simulink model "perturbacion2"  (R2018b)
settings: Solver=VariableStepAuto  StartTime=0.0  StopTime=10.0  RelTol=1e-3
undefined symbols (not defined in the file): AHat, BHat, CHat, DHat, FHat, K, Kgain, Tao
settings Model: Creator=AlfredoMaussa  LastModifiedBy=AlfredoMaussa
settings SolverCC: ZeroCrossAlgorithm=Adaptive
settings DebuggingCC: IgnoredZcDiagnostic=none

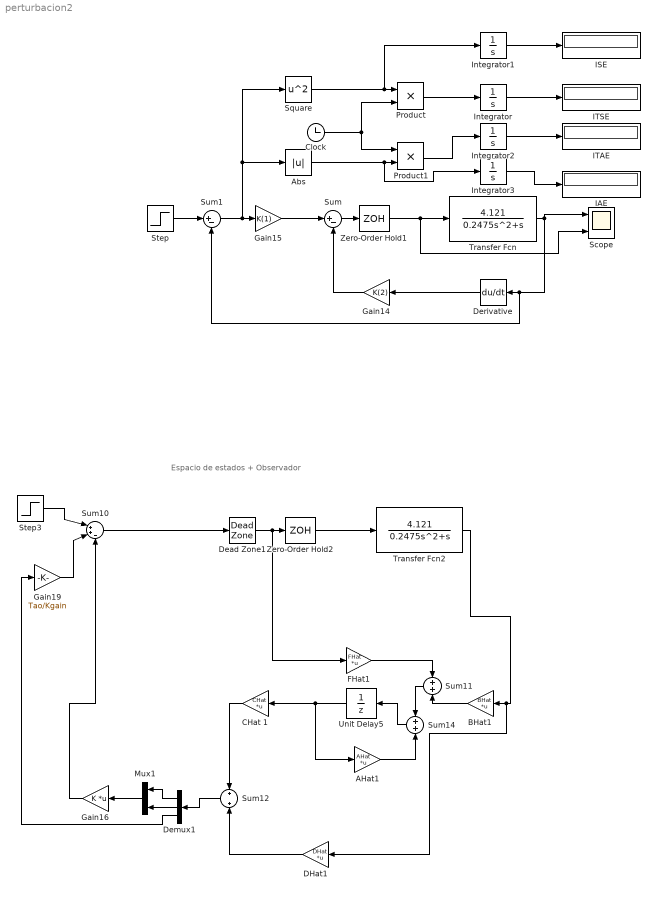
== system perturbacion2 ==
  note: Espacio de estados + Observador
  AHat1 : Gain  Gain=AHat  Multiplication=Matrix(K*u)
  Abs : Abs
  BHat1 : Gain  Gain=BHat  Multiplication=Matrix(K*u)
  CHat 1 : Gain  Gain=CHat  Multiplication=Matrix(K*u)
  Clock : Clock
  DHat1 : Gain  Gain=DHat  Multiplication=Matrix(K*u)
  Dead Zone1 : DeadZone  LowerValue=0  UpperValue=0  SaturateOnIntegerOverflow=on
  Demux1 : Demux  Outputs=3
  Derivative : Derivative  CoefficientInTFapproximation=100
  FHat1 : Gain  Gain=FHat  Multiplication=Matrix(K*u)
  Gain14 : Gain  Gain=K(2)
  Gain15 : Gain  Gain=K(1)
  Gain16 : Gain  Gain=K  Multiplication=Matrix(K*u)
  Gain19 : Gain  Gain=Tao/Kgain
  IAE : Display
  ISE : Display
  ITAE : Display
  ITSE : Display
  Integrator{,1..3} (4 alike) : Integrator
  Mux1 : Mux  Inputs=2
  Product : Product
  Product1 : Product
  Scope : Scope  NumInputPorts=2
  Square : Math  Operator=square  SaturateOnIntegerOverflow=on
  Step : Step  Time=0  SampleTime=0
  Step3 : Step  Time=0  SampleTime=0
  Sum : Sum  Inputs=|+-
  Sum1 : Sum  Inputs=|+-
  Sum10 : Sum  Inputs=|++-
  Sum11 : Sum  Inputs=+|+
  Sum12 : Sum  Inputs=+||+
  Sum14 : Sum  Inputs=+|+
  Transfer Fcn : TransferFcn  Numerator=[4.121]  Denominator=[0.2475 1 0]
  Transfer Fcn2 : TransferFcn  Numerator=[4.121]  Denominator=[0.2475 1 0]
  Unit Delay5 : UnitDelay  InitialCondition=[0,0]  SampleTime=0.005
  Zero-Order Hold1 : ZeroOrderHold  SampleTime=0.005
  Zero-Order Hold2 : ZeroOrderHold  SampleTime=0.005
  wires:
  Gain15/1 -> Sum/1
  Mux1/1 -> Gain16/1
  CHat 1/1 -> Sum12/1
  Step3/1 -> Sum10/1
  Unit Delay5/1 -> CHat 1/1, AHat1/1
  Sum11/1 -> Sum14/1
  FHat1/1 -> Sum11/1
  BHat1/1 -> Sum11/2
  Sum14/1 -> Unit Delay5/1
  DHat1/1 -> Sum12/2
  Derivative/1 -> Gain14/1
  Sum1/1 -> Square/1, Abs/1, Gain15/1
  Sum12/1 -> Demux1/1
  Demux1/1 -> Mux1/1
  Step/1 -> Sum1/1
  Sum/1 -> Zero-Order Hold1/1
  Demux1/2 -> Mux1/2
  Gain14/1 -> Sum/2
  Transfer Fcn/1 -> Sum1/2, Derivative/1, Scope/1
  AHat1/1 -> Sum14/2
  Zero-Order Hold1/1 -> Scope/2, Transfer Fcn/1
  Demux1/3 -> Gain19/1
  Zero-Order Hold2/1 -> Transfer Fcn2/1
  Transfer Fcn2/1 -> DHat1/1, BHat1/1
  Sum10/1 -> Dead Zone1/1
  Dead Zone1/1 -> FHat1/1, Zero-Order Hold2/1
  Gain16/1 -> Sum10/3
  Gain19/1 -> Sum10/2
  Clock/1 -> Product1/1, Product/2
  Square/1 -> Integrator1/1, Product/1
  Abs/1 -> Integrator3/1, Product1/2
  Product/1 -> Integrator/1
  Product1/1 -> Integrator2/1
  Integrator1/1 -> ISE/1
  Integrator/1 -> ITSE/1
  Integrator2/1 -> ITAE/1
  Integrator3/1 -> IAE/1
